simulink model "gm_echo"  (R2024a)
settings: Solver=VariableStepAuto  StartTime=0.0  StopTime=20  RelTol=1e-3
settings Model: Creator=fermata  LastModifiedBy=fermata
settings OptimizationCC: BlockReduction=off  ConditionallyExecuteInputs=off
settings DebuggingCC: InheritedTsInSrcMsg=none

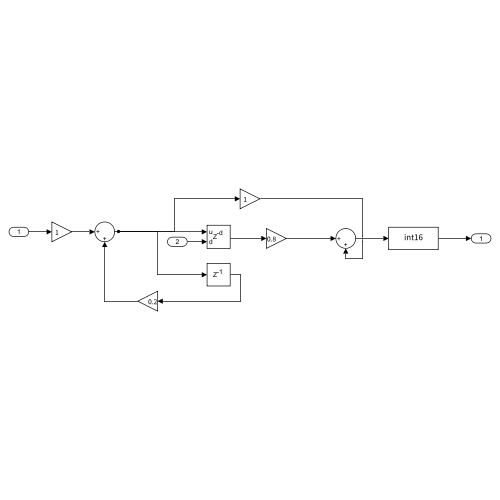
[thumbnail: Simulink's stored preview of the top-level diagram]
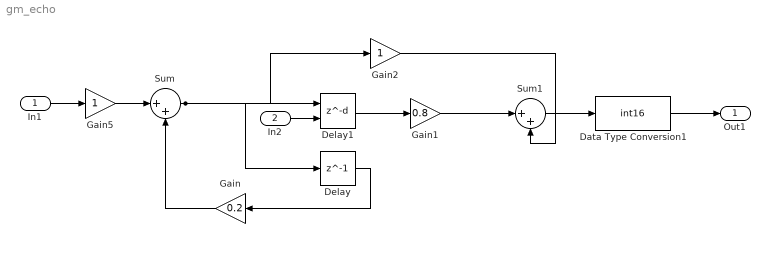
== system gm_echo ==
  In1 : Inport  OutDataTypeStr=int16  PortDimensions=1  SampleTime=0.4
  In2 : Inport  Port=2  OutDataTypeStr=uint32  PortDimensions=1  SampleTime=0.4
  Data Type Conversion1 : DataTypeConversion  OutDataTypeStr=int16  SaturateOnIntegerOverflow=off  RndMeth=Floor
  Delay : Delay  DelayLength=1  InitialCondition=0
  Delay1 : Delay  DelayLengthSource=Input port  DelayLength=1  DelayLengthUpperLimit=1024  InitialCondition=0
      settings: InputPortMap=u0,p1
  Gain : Gain  Gain=0.2  OutDataTypeStr=fixdt(1, 32, 14)  RndMeth=Simplest  SaturateOnIntegerOverflow=on
  Gain1 : Gain  Gain=0.8  OutDataTypeStr=fixdt(1, 64, 45)
  Gain2 : Gain  OutDataTypeStr=fixdt(1, 64, 44)
  Gain5 : Gain  OutDataTypeStr=fixdt(1, 32, 14)
  Sum : Sum  Inputs=|++  OutDataTypeStr=fixdt(1, 32, 14)
  Sum1 : Sum  Inputs=|++  OutDataTypeStr=fixdt(1, 64, 44)
  Out1 : Outport  OutDataTypeStr=int16  SampleTime=0.4
  wires:
  In1/1 -> Gain5/1
  In2/1 -> Delay1/2
  Data Type Conversion1/1 -> Out1/1
  Delay/1 -> Gain/1
  Delay1/1 -> Gain1/1
  Gain/1 -> Sum/2
  Gain1/1 -> Sum1/1
  Gain2/1 -> Sum1/2
  Gain5/1 -> Sum/1
  Sum/1 -> Gain2/1, Delay1/1, Delay/1
  Sum1/1 -> Data Type Conversion1/1
